simulink model "Motion_Planning"  (R2021a)
settings: Solver=FixedStepDiscrete  StartTime=0.0  StopTime=inf  FixedStep=1  RelTol=1e-3
model workspace (MAT data in the model file):
  SL_ROS_VariableLengthArrays_MaxSizes.CommonInfo.ArrayTruncateAction = 'EmitWarning'
  SL_ROS_VariableLengthArrays_MaxSizes.MsgTypeMap = containers.Map
  SL_ROS_VariableLengthArrays_MaxSizes.MsgTypeMap.serialization.keys = {'geometry_msgs/PoseArray', 'std_msgs/Float32MultiArray'}
  SL_ROS_VariableLengthArrays_MaxSizes.MsgTypeMap.serialization.values{1}.PropertyName = 'Poses'
  SL_ROS_VariableLengthArrays_MaxSizes.MsgTypeMap.serialization.values{1}.DataType = 'geometry_msgs/Pose'
  SL_ROS_VariableLengthArrays_MaxSizes.MsgTypeMap.serialization.values{1}.MaxLength = 100
  SL_ROS_VariableLengthArrays_MaxSizes.MsgTypeMap.serialization.values{2}.PropertyName = 'Data'
  SL_ROS_VariableLengthArrays_MaxSizes.MsgTypeMap.serialization.values{2}.DataType = 'single'
  SL_ROS_VariableLengthArrays_MaxSizes.MsgTypeMap.serialization.values{2}.MaxLength = 2004
  SL_ROS_VariableLengthArrays_MaxSizes.MsgTypeMap.serialization.uniformity = 0
  SL_ROS_VariableLengthArrays_MaxSizes.MsgTypeMap.serialization.keyType = 'char'
  SL_ROS_VariableLengthArrays_MaxSizes.MsgTypeMap.serialization.valueType = 'any'
undefined symbols (not defined in the file): Data, Data_SL_Info
libraries: robotlib x5, simulink_extras x2
settings Model: EnablePacing=on  OrderedModelArguments=off  ExplicitPartitioning=on  Creator=HS  LastModifiedBy=xhu-fsac
settings SolverCC: ZeroCrossAlgorithm=Adaptive  AlgebraicLoopSolver=TrustRegion
settings DataIOCC: ReturnWorkspaceOutputs=off
settings OptimizationCC: EnhancedBackFolding=on  PassReuseOutputArgsAs=Individual arguments  ZeroExternalMemoryAtStartup=off  ZeroInternalMemoryAtStartup=off  MaxStackSize=64  OptimizeBlockOrder=speed  DifferentSizesBufferReuse=on  OptimizationCustomize=off  EfficientTunableParamExpr=on
settings DebuggingCC: IgnoredZcDiagnostic=none  ParameterTunabilityLossMsg=error  SFMachineParentedDataDiag=warning
settings HardwareCC: ProdBitPerPointer=32  ProdBitPerSizeT=32  ProdBitPerPtrDiffT=32  ProdLargestAtomicFloat=None  ProdIntDivRoundTo=Undefined  ProdEndianess=Unspecified  ProdWordSize=32  ProdHWDeviceType=Generic->Unspecified (assume 32-bit Generic)
settings RTWCC: SystemTargetFile=ert.tlc  HardwareBoard=Robot Operating System (ROS)  TLCOptions="-aInlineSetEventsForThisBaseRateFcn=TLC_FALSE -aSuppressMultiTaskScheduler=TLC_FALSE  -aRateBasedStepFcn=0"  TemplateMakefile=ert_default_tmf  Toolchain=Catkin  TargetLang=C++
settings CodeAppCC: ForceParamTrailComments=on  IgnoreCustomStorageClasses=off  OperatorAnnotations=on  SimulinkDataObjDesc=on  SFDataObjDesc=on  InsertBlockDesc=on
settings ERTTargetCC: SupportVariableSizeSignals=on

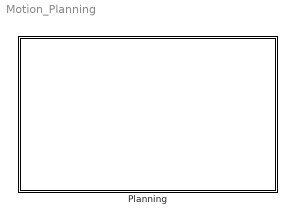
== system Motion_Planning ==
  Planning : Subsystem  TreatAsAtomicUnit=on  SystemSampleTime=1

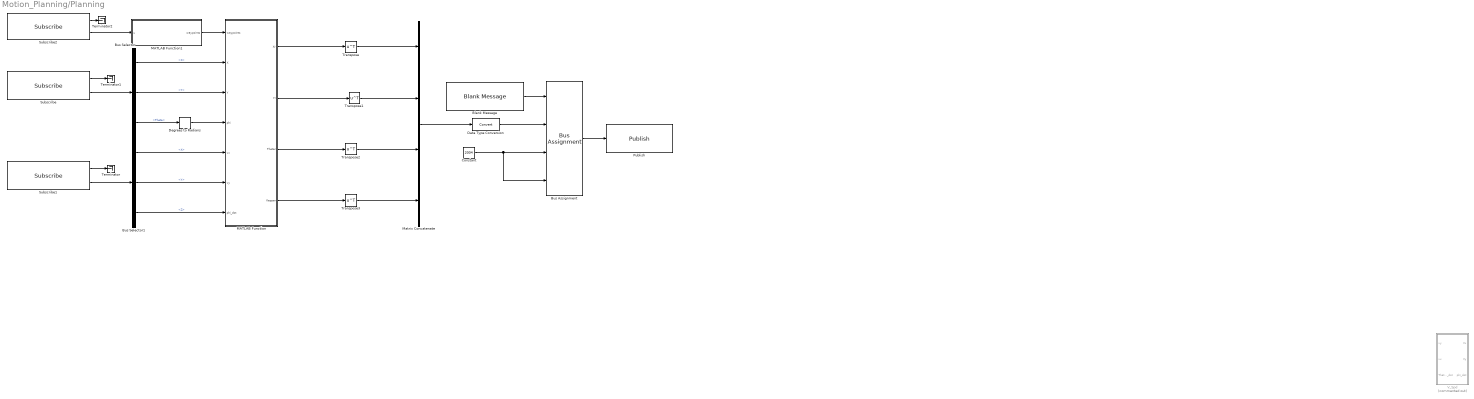
== system Motion_Planning/Planning ==
  Blank Message : robotlib/Blank Message  messageClass=Message  entityType=std_msgs/Float32MultiArray  messageType=std_msgs/Float32MultiArray  SampleTime=inf  legacyBusStruct=off
  Bus Assignment : BusAssignment  AssignedSignals=Data,Data_SL_Info.CurrentLength,Data_SL_Info.ReceivedLength
  Bus Selector : BusSelector  OutputSignals=X,Y,Theta
  Bus Selector1 : BusSelector  OutputSignals=Linear.X,Linear.Y,Linear.Z
  Constant : Constant  Value=2004  OutDataTypeStr=uint32
  Data Type Conversion : DataTypeConversion
  Degrees to Radians : simulink_extras/Transformations/Degrees to Radians
  MATLAB Function : MATLAB Function  TreatAsAtomicUnit=on
  MATLAB Function1 : MATLAB Function  TreatAsAtomicUnit=on
  Matrix Concatenate : Concatenate  NumInputs=4  ConcatenateDimension=2
  Publish : robotlib/Publish  topicSource=Specify your own  topic=/Planning_Trajectory  messageType=std_msgs/Float32MultiArray  legacyBusStruct=off  messageQueueLength=1
  Subscribe : robotlib/Subscribe  topicSource=Specify your own  topic=/canalystii_ros/vehicle_Pose  messageType=geometry_msgs/Pose2D  SampleTime=-1  legacyBusStruct=off  messageQueueLength=1
  Subscribe1 : robotlib/Subscribe  topicSource=Specify your own  topic=/canalystii_ros/vehicle_spd  messageType=geometry_msgs/Twist  SampleTime=-1  legacyBusStruct=off  messageQueueLength=1
  Subscribe2 : robotlib/Subscribe  topicSource=Specify your own  topic=/point  messageType=geometry_msgs/PoseArray  SampleTime=-1  legacyBusStruct=off  messageQueueLength=1
  Terminator : Terminator
  Terminator1 : Terminator
  Terminator2 : Terminator
  Transpose{,1..3} (4 alike) : Math  Operator=transpose  SaturateOnIntegerOverflow=on
  V_Spd : Subsystem  Commented=on
  wires:
  Bus Selector1/3 -> MATLAB Function/7(phi_dot)  "<Z>"
  Subscribe/2 -> Bus Selector/1
  Subscribe1/2 -> Bus Selector1/1
  Transpose/1 -> Matrix Concatenate/1
  Bus Selector/1 -> MATLAB Function/2(X)  "<X>"
  Bus Selector1/2 -> MATLAB Function/6(vy)  "<Y>"
  Bus Assignment/1 -> Publish/1
  Bus Selector/2 -> MATLAB Function/3(Y)  "<Y>"
  MATLAB Function/1(Xr) -> Transpose/1
  Bus Selector1/1 -> MATLAB Function/5(vx)  "<X>"
  MATLAB Function/3(Thetar) -> Transpose2/1
  Transpose3/1 -> Matrix Concatenate/4
  Subscribe/1 -> Terminator1/1
  Transpose1/1 -> Matrix Concatenate/2
  Blank Message/1 -> Bus Assignment/1
  Data Type Conversion/1 -> Bus Assignment/2
  Degrees to Radians/1 -> MATLAB Function/4(phi)
  Constant/1 -> Bus Assignment/4, Bus Assignment/3
  Subscribe1/1 -> Terminator/1
  Matrix Concatenate/1 -> Data Type Conversion/1
  Bus Selector/3 -> Degrees to Radians/1  "<Theta>"
  MATLAB Function/2(Yr) -> Transpose1/1
  Transpose2/1 -> Matrix Concatenate/3
  MATLAB Function/4(Kappar) -> Transpose3/1
  Subscribe2/2 -> MATLAB Function1/1(u)
  MATLAB Function1/1(waypoints) -> MATLAB Function/1(waypoints)
  Subscribe2/1 -> Terminator2/1

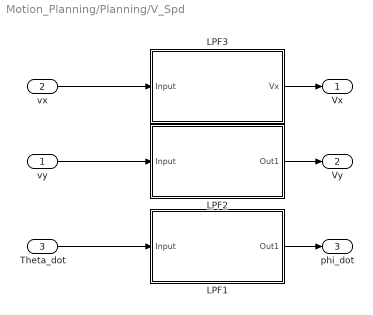
== system Motion_Planning/Planning/V_Spd ==
  vy : Inport
  vx : Inport  Port=2
  Theta_dot : Inport  Port=3
  LPF1 : Subsystem  TreatAsAtomicUnit=on
  LPF2 : Subsystem  TreatAsAtomicUnit=on
  LPF3 : Subsystem  TreatAsAtomicUnit=on
  Vx : Outport  VectorParamsAs1DForOutWhenUnconnected=off
  Vy : Outport  Port=2  VectorParamsAs1DForOutWhenUnconnected=off
  phi_dot : Outport  Port=3  VectorParamsAs1DForOutWhenUnconnected=off
  wires:
  Theta_dot/1 -> LPF1/1(Input)
  LPF1/1(Out1) -> phi_dot/1
  LPF2/1(Out1) -> Vy/1
  LPF3/1(Vx) -> Vx/1
  vx/1 -> LPF3/1(Input)
  vy/1 -> LPF2/1(Input)

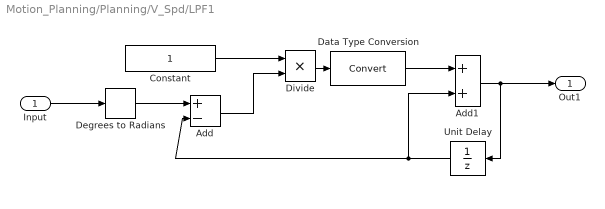
== system Motion_Planning/Planning/V_Spd/LPF1 ==
  Input : Inport
  Add : Sum  Inputs=+-
  Add1 : Sum
  Constant : Constant
  Data Type Conversion : DataTypeConversion
  Degrees to Radians : simulink_extras/Transformations/Degrees to Radians
  Divide : Product  Inputs=**
  Unit Delay : UnitDelay  SampleTime=-1  HasFrameUpgradeWarning=on
  Out1 : Outport  VectorParamsAs1DForOutWhenUnconnected=off
  wires:
  Divide/1 -> Data Type Conversion/1
  Input/1 -> Degrees to Radians/1
  Constant/1 -> Divide/1
  Add/1 -> Divide/2
  Data Type Conversion/1 -> Add1/1
  Add1/1 -> Unit Delay/1, Out1/1
  Unit Delay/1 -> Add/2, Add1/2
  Degrees to Radians/1 -> Add/1

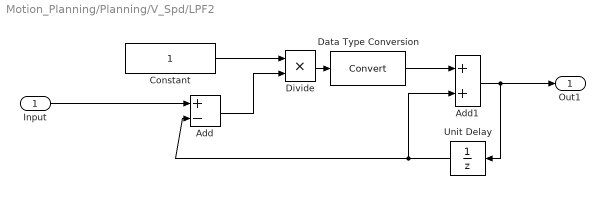
== system Motion_Planning/Planning/V_Spd/LPF2 ==
  Input : Inport
  Add : Sum  Inputs=+-
  Add1 : Sum
  Constant : Constant
  Data Type Conversion : DataTypeConversion
  Divide : Product  Inputs=**
  Unit Delay : UnitDelay  SampleTime=-1  HasFrameUpgradeWarning=on
  Out1 : Outport  VectorParamsAs1DForOutWhenUnconnected=off
  wires:
  Divide/1 -> Data Type Conversion/1
  Constant/1 -> Divide/1
  Add/1 -> Divide/2
  Data Type Conversion/1 -> Add1/1
  Add1/1 -> Unit Delay/1, Out1/1
  Unit Delay/1 -> Add/2, Add1/2
  Input/1 -> Add/1

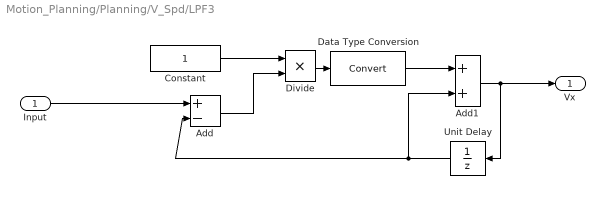
== system Motion_Planning/Planning/V_Spd/LPF3 ==
  Input : Inport
  Add : Sum  Inputs=+-
  Add1 : Sum
  Constant : Constant
  Data Type Conversion : DataTypeConversion
  Divide : Product  Inputs=**
  Unit Delay : UnitDelay  SampleTime=-1  HasFrameUpgradeWarning=on
  Vx : Outport  VectorParamsAs1DForOutWhenUnconnected=off
  wires:
  Input/1 -> Add/1
  Unit Delay/1 -> Add1/2, Add/2
  Add1/1 -> Vx/1, Unit Delay/1
  Data Type Conversion/1 -> Add1/1
  Add/1 -> Divide/2
  Constant/1 -> Divide/1
  Divide/1 -> Data Type Conversion/1

== matlab function Motion_Planning/Planning/MATLAB Function1 ==
  data: u input; waypoints output size=[100,2] [..100]
function waypoints = fcn(u)
len = u.Poses_SL_Info.ReceivedLength;
waypoint = zeros(100,2);
waypoints = zeros(100,2);
for i = 1:len
    waypoint(i,1) = u.Poses(i).Position.X;
    waypoint(i,2) = u.Poses(i).Position.Y;
end
[row,~] = size(waypoint);
for j = 1:row
    if waypoint(j,1) == 0
        waypoints = waypoint(1:j-1,1:2);
        break;
    end
end

end

== matlab function Motion_Planning/Planning/MATLAB Function ==
  data: waypoints input size=[100,2] [..100]; X input size=1; Y input size=1; phi input size=1; vx input size=1; vy input size=1; phi_dot input size=1; Xr output; Yr output; Thetar output; Kappar output
function [Xr,Yr,Thetar,Kappar] = fcn( waypoints, X, Y,  phi,vx, vy,phi_dot)
TrajGlobal =zeros(501,6);
Xr = zeros(501,1);
Yr = zeros(501,1);
Thetar = zeros(501,1);
Kappar = zeros(501,1);
% Obs_pos =zeros(1,6);
vehicle_pose_frenet_s_ref = zeros(1,6);
diff_sr = zeros(501,1);

persistent  planning_flag last_frenet_trajectory 
 
refPath = referencePathFrenet(waypoints,'DiscretizationDistance',0.01);

connector = trajectoryGeneratorFrenet(refPath,'TimeResolution',0.01);


if isempty(planning_flag)
    planning_flag = 0;
end
if isempty(last_frenet_trajectory)
    last_frenet_trajectory = zeros(501,6);
end

%把车辆全局坐标系转换到frenet下
v = sqrt(vx^2 + vy^2);
if v <= 0.1
    v = 0.1;
    kappa = 0;
else
    kappa = phi_dot/v;
end

%%%%将车辆的位置转换成frenet坐标系下面
%如果第一次规划就用车辆起始位置
%如果另外的规划，则用上一次车辆投影点的轨迹作为起始轨迹
vehicle_pose = [X,Y,phi,kappa,v,0];
vehicle_pose_frenet_s = global2frenet(refPath,vehicle_pose);
vehicle_pose_frenet_s(2) = 3;
vehicle_pose_frenet_s(3) = 0;
vehicle_pose_frenet_s(4) = 0;
vehicle_pose_frenet_s(5) = 0;
vehicle_pose_frenet_s(6) = 0;


vehicle_pose_frenet_e = vehicle_pose_frenet_s;
vehicle_pose_frenet_e(1) = vehicle_pose_frenet_e(1) + 10;
vehicle_pose_frenet_e(2) = 3;
vehicle_pose_frenet_e(3) = 0;
vehicle_pose_frenet_e(4) = 0;
vehicle_pose_frenet_e(5) = 0;
vehicle_pose_frenet_e(6) = 0;

if planning_flag == 0 %第一次规划 
    %用自车起始位置
    vehicle_pose_frenet_s_ref(:) = vehicle_pose_frenet_s(:); 
    
    planning_flag = 1;   
elseif planning_flag == 1 %其他规划
    %用上一次车辆投影点的位置拼接轨迹
    %找车辆最近点的索引
    diff_sr(:) = abs(last_frenet_trajectory(:,1) - vehicle_pose_frenet_s(1));
    [~,index] = min(diff_sr);
    vehicle_pose_frenet_s_ref(:) = last_frenet_trajectory(index,:);
end


%%%%生成全局坐标系
[newTrajFrenet_noCol,newTrajGlobal_noCol] = connect(connector,vehicle_pose_frenet_s_ref,vehicle_pose_frenet_e,5);
TrajGlobal(:,:) = newTrajGlobal_noCol.Trajectory(:,:);
Xr(:) = TrajGlobal(:,1);
Yr(:) = TrajGlobal(:,2);
Thetar(:) = TrajGlobal(:,3);
Kappar(:) = TrajGlobal(:,4);

% %%%%添加车辆自身
% obsList = dynamicCapsuleList;
% obsList.MaxNumSteps = 501;
% egoID1 = 1;
% geom = struct("Length",3.7,"Radius",0.9,"FixedTransform",eye(3));
% states = zeros(length(Xr),3);
% states(:,1) = Xr;
% states(:,2) = Yr;
% states(:,3) = Thetar;
% egoCapsule = struct('ID',egoID1,'States',states,'Geometry',geom);
% addEgo(obsList,egoCapsule);

%%%%添加障碍物
% Obs_pos(:) = [obs_s 0 0 obs_l 0 0];
% Obs_pos_global = frenet2global(refPath,Obs_pos);
% obsState = zeros(1,3);
% obsState(1,1) = Obs_pos_global(1);
% obsState(1,2) = Obs_pos_global(2); 
% obsState(1,3) = Obs_pos_global(3);
% obsCapsule = struct('ID',1,'States',obsState,'Geometry',geom);
% addObstacle(obsList,obsCapsule);
% collisions = zeros(1,501);
% collisions(:,:) = checkCollision(obsList)';

% if any(collisions)
%     vehicle_pose_frenet_e = vehicle_pose_frenet_s;
%     vehicle_pose_frenet_e(1) = vehicle_pose_frenet_e(1) + 20;
%     vehicle_pose_frenet_e(2) = 3;
%     vehicle_pose_frenet_e(3) = 0;
%     vehicle_pose_frenet_e(4) = 0;%%%%轨迹往左还是右偏
%     vehicle_pose_frenet_e(5) = 0;
%     vehicle_pose_frenet_e(6) = 0;
%     
%     [newTrajFrenet_hasCol,newTrajGlobal_hasCol] = connect(connector,vehicle_pose_frenet_s_ref,vehicle_pose_frenet_e,5);
%     TrajGlobal(:,:) = newTrajGlobal_hasCol.Trajectory(:,:);
%     Xr(:) = TrajGlobal(:,1);
%     Yr(:) = TrajGlobal(:,2);
%     Thetar(:) = TrajGlobal(:,3);
%     Kappar(:) = TrajGlobal(:,4);
%     
%     last_frenet_trajectory(:) = newTrajFrenet_hasCol.Trajectory(:,:);  
% else

last_frenet_trajectory(:) = newTrajFrenet_noCol.Trajectory(:,:);  



Plot();
% 
% 
% 
% 
function Plot()
%     
coder.extrinsic('delete');
coder.extrinsic('plot');
figure(2);
[minxval,~] = min(waypoints(:,1));
[maxxval,~] = max(waypoints(:,1));
[minyval,~] = min(waypoints(:,2));
[maxyval,~] = max(waypoints(:,2));
axis([minxval-5,maxxval+5,minyval-5,maxyval+5],'equal');
 persistent h 
 if isempty(h)
    h = plot(Xr,Yr,'w');  
 end
 delete(h);
 plot(waypoints(:,1),waypoints(:,2),'r.');%%%%参考轨迹
 hold on;
%  show(refPath,'Parent');
%  rectangle('Position',[obsState(1,1)-0.9, obsState(1,2) - 0.9, 1.8, 1.8]...
%      ,'Curvature',[1,1]);
%    hold on;

 h = plot(Xr,Yr,'g');%%%拟合轨迹

plot(X,Y,'ko');%%%车辆
hold on;
% 

end

end
